simulink model "Simulation_in_Simulink"  (R2021b)
settings: Solver=FixedStepAuto  StartTime=0.0  StopTime=10  FixedStep=0.02  RelTol=1e-3
(part 1 of 5)
settings Model: Creator=sadegh  LastModifiedBy=sadegh

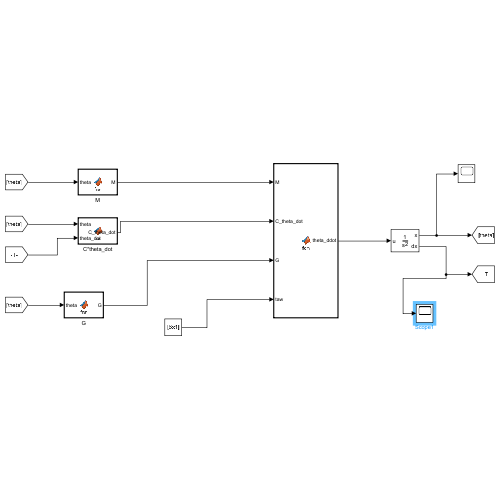
[thumbnail: Simulink's stored preview of the top-level diagram]
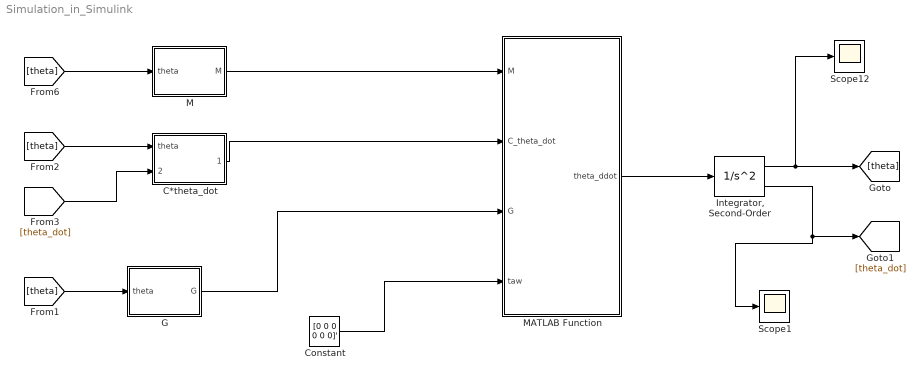
== system Simulation_in_Simulink ==
  C*theta_dot : MATLAB Function  TreatAsAtomicUnit=on
  Constant : Constant  Value=[0 0 0 0 0 0]'
  G : MATLAB Function  TreatAsAtomicUnit=on
  "Integrator, Second-Order" : SecondOrderIntegrator  ICDXDT=zeros(6,1)
  M : MATLAB Function  TreatAsAtomicUnit=on
  MATLAB Function : MATLAB Function  TreatAsAtomicUnit=on
  Scope1 : Scope
  Scope12 : Scope
  wires:
  MATLAB Function/1(theta_ddot) -> "Integrator, Second-Order"/1
  "Integrator, Second-Order"/1 -> Scope12/1, [theta]
  "Integrator, Second-Order"/2 -> Scope1/1, [theta_dot]
  [theta] -> G/1(theta)
  [theta] -> C*theta_dot/1(theta)
  [theta_dot] -> C*theta_dot/2(theta_dot)
  M/1(M) -> MATLAB Function/1(M)
  G/1(G) -> MATLAB Function/3(G)
  Constant/1 -> MATLAB Function/4(taw)
  C*theta_dot/1(C_theta_dot) -> MATLAB Function/2(C_theta_dot)
  [theta] -> M/1(theta)
